simulink model "Control1"  (R2015a)
settings: Solver=ode45  SolverMode=SingleTasking  StartTime=0.0  StopTime=500  RelTol=1e-3
InitFcn:
  | clear all
StopFcn:
  | figure(1)
  | plot(energy)
  | xlabel('Time (s)')
  | ylabel('Energy Extracted (Jules)')
  | title('Energy Extracted')
settings Model: Creator=Piyush  LastModifiedBy=Piyush
settings OptimizationCC: BlockReduction=off  BooleanDataType=off
settings DebuggingCC: SaveWithParameterizedLinksMsg=none  UnderspecifiedInitializationDetection=Classic  MergeDetectMultiDrivingBlocksExec=none  SignalResolutionControl=TryResolveAllWithWarning
settings HardwareCC: TargetUnknown=on

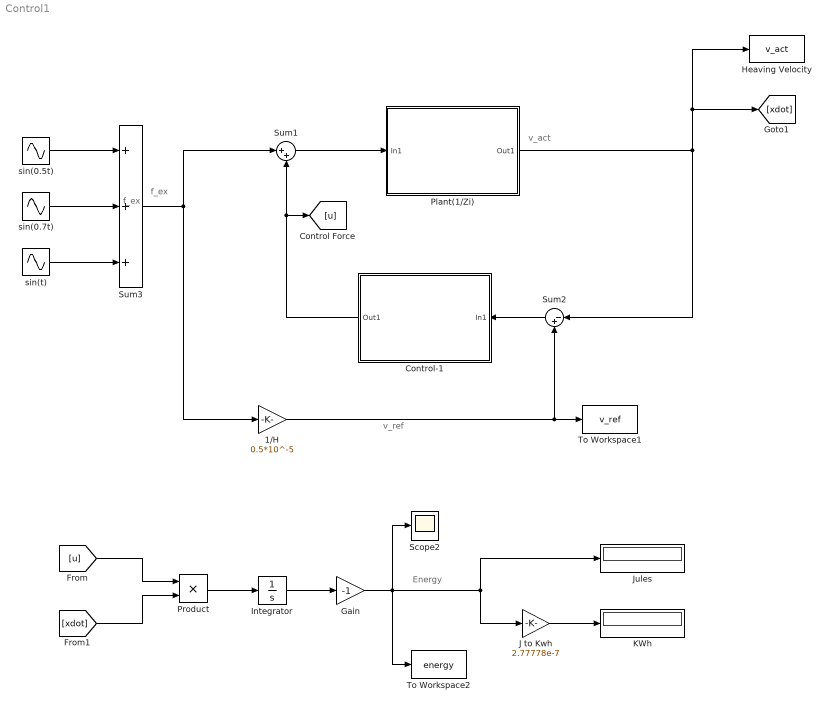
== system Control1 ==
  note: Energy
  note: f_ex
  note: v_act
  note: v_ref
  note: f_ex
  1/H : Gain  Gain=0.5*10^-5
  Control-1 : Subsystem
  Gain : Gain  Gain=-1
  Heaving Velocity : ToWorkspace  VariableName=v_act  SaveFormat=Timeseries  SampleTime=-1
  Integrator : Integrator  ZeroCross=off
  J to Kwh : Gain  Gain=2.77778e-7
  Jules : Display
  KWh : Display
  Plant(1/Zi) : Subsystem
  Product : Product
  Scope2 : Scope
      settings: TimeRange=100  YMin=1.89e+09  YMax=2.05e+09  SaveName=ScopeData2
  Sum1 : Sum  Inputs=|++
  Sum2 : Sum  Inputs=|-+
  Sum3 : Sum  Inputs=+++
  To Workspace1 : ToWorkspace  VariableName=v_ref  SaveFormat=Timeseries  SampleTime=-1
  To Workspace2 : ToWorkspace  VariableName=energy  SaveFormat=Timeseries  SampleTime=-1
  sin(0.5t) : Sin  Amplitude=5*10^5  Frequency=.5  SampleTime=0
  sin(0.7t) : Sin  Amplitude=5*10^5  Frequency=.7  SampleTime=0
  sin(t) : Sin  Amplitude=5*10^5  SampleTime=0
  wires:
  [u] -> Product/1
  [xdot] -> Product/2
  Product/1 -> Integrator/1
  Integrator/1 -> Gain/1
  Gain/1 -> J to Kwh/1, Jules/1, To Workspace2/1, Scope2/1
  Sum1/1 -> Plant(1/Zi)/1(In1)
  Control-1/1(Out1) -> Sum1/2, [u]
  Sum2/1 -> Control-1/1(In1)
  Sum3/1 -> Sum1/1, 1/H/1
  1/H/1 -> To Workspace1/1, Sum2/2
  Plant(1/Zi)/1(Out1) -> Heaving Velocity/1, [xdot], Sum2/1
  J to Kwh/1 -> KWh/1
  sin(0.5t)/1 -> Sum3/1
  sin(0.7t)/1 -> Sum3/2
  sin(t)/1 -> Sum3/3

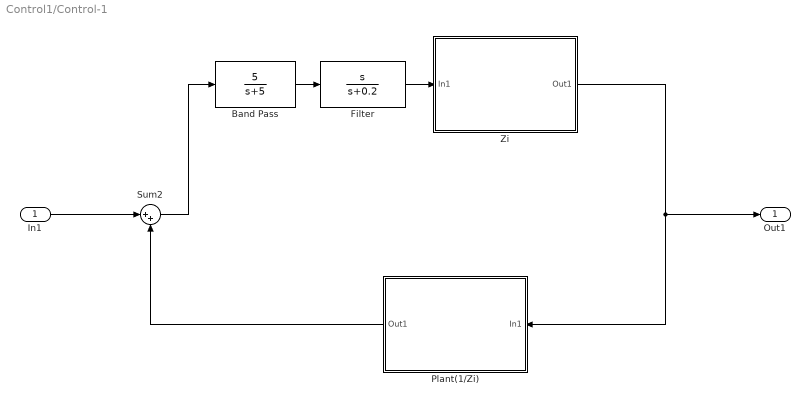
== system Control1/Control-1 ==
  In1 : Inport
  Band Pass : TransferFcn  Numerator=[5]  Denominator=[1 5]
  Filter : TransferFcn  Numerator=[1 0]  Denominator=[1 0.2]
  Plant(1/Zi) : Subsystem
  Sum2 : Sum  Inputs=|++
  Zi : Subsystem
  Out1 : Outport
  wires:
  In1/1 -> Sum2/1
  Band Pass/1 -> Filter/1
  Sum2/1 -> Band Pass/1
  Zi/1(Out1) -> Plant(1/Zi)/1(In1), Out1/1
  Filter/1 -> Zi/1(In1)
  Plant(1/Zi)/1(Out1) -> Sum2/2

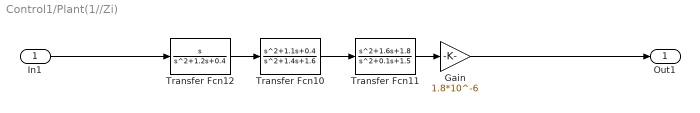
== system Control1/Plant(1//Zi) ==
  In1 : Inport
  Gain : Gain  Gain=1.8*10^-6
  Transfer Fcn10 : TransferFcn  Numerator=[1 1.1 0.4]  Denominator=[1 1.4 1.6]
  Transfer Fcn11 : TransferFcn  Numerator=[1 1.6 1.8]  Denominator=[1 0.1 1.5]
  Transfer Fcn12 : TransferFcn  Numerator=[1 0]  Denominator=[1 1.2 0.4]
  Out1 : Outport
  wires:
  In1/1 -> Transfer Fcn12/1
  Transfer Fcn11/1 -> Gain/1
  Transfer Fcn12/1 -> Transfer Fcn10/1
  Transfer Fcn10/1 -> Transfer Fcn11/1
  Gain/1 -> Out1/1

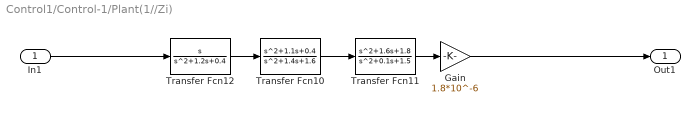
== system Control1/Control-1/Plant(1//Zi) ==
  In1 : Inport
  Gain : Gain  Gain=1.8*10^-6
  Transfer Fcn10 : TransferFcn  Numerator=[1 1.1 0.4]  Denominator=[1 1.4 1.6]
  Transfer Fcn11 : TransferFcn  Numerator=[1 1.6 1.8]  Denominator=[1 0.1 1.5]
  Transfer Fcn12 : TransferFcn  Numerator=[1 0]  Denominator=[1 1.2 0.4]
  Out1 : Outport
  wires:
  In1/1 -> Transfer Fcn12/1
  Transfer Fcn11/1 -> Gain/1
  Transfer Fcn12/1 -> Transfer Fcn10/1
  Transfer Fcn10/1 -> Transfer Fcn11/1
  Gain/1 -> Out1/1

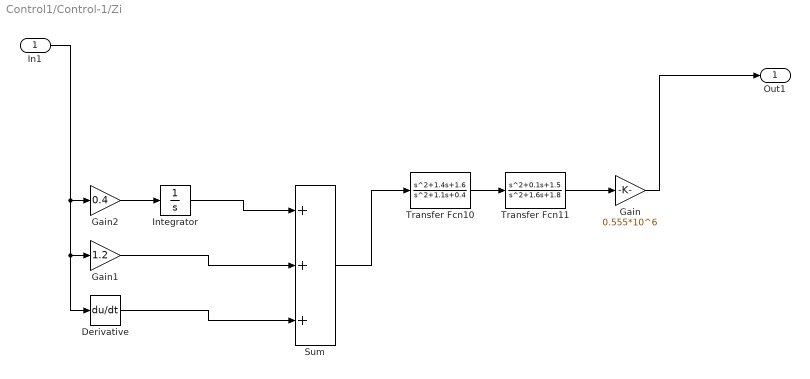
== system Control1/Control-1/Zi ==
  In1 : Inport
  Derivative : Derivative
  Gain : Gain  Gain=0.555*10^6
  Gain1 : Gain  Gain=1.2
  Gain2 : Gain  Gain=0.4
  Integrator : Integrator
  Sum : Sum  Inputs=+++
  Transfer Fcn10 : TransferFcn  Numerator=[1 1.4 1.6]  Denominator=[1 1.1 0.4]
  Transfer Fcn11 : TransferFcn  Numerator=[1 0.1 1.5]  Denominator=[1 1.6 1.8]
  Out1 : Outport
  wires:
  Gain/1 -> Out1/1
  Transfer Fcn10/1 -> Transfer Fcn11/1
  Transfer Fcn11/1 -> Gain/1
  In1/1 -> Gain2/1, Derivative/1, Gain1/1
  Sum/1 -> Transfer Fcn10/1
  Derivative/1 -> Sum/3
  Gain1/1 -> Sum/2
  Gain2/1 -> Integrator/1
  Integrator/1 -> Sum/1
